simulink subsystem "Throttle_Map_2WD_NO_FILTER_NO_REGEN"  (R2023b)
settings: Solver=VariableStepAuto  StartTime=0.0  StopTime=10.0  RelTol=1e-3
undefined symbols (not defined in the file): tvs
settings Model: Creator=Inver  LastModifiedBy=Inver

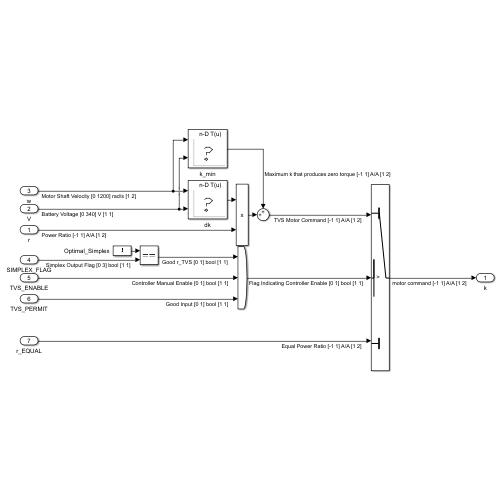
[thumbnail: Simulink's stored preview of the top-level diagram]
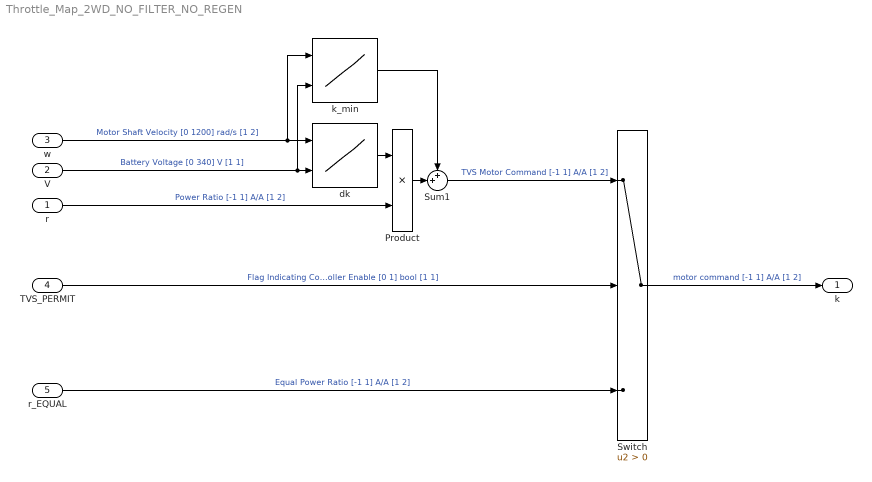
== system Throttle_Map_2WD_NO_FILTER_NO_REGEN ==
  r : Inport
  V : Inport  Port=2
  w : Inport  Port=3
  TVS_PERMIT : Inport  Port=4
  r_EQUAL : Inport  Port=5
  Product : Product
  Sum1 : Sum  Inputs=++|
  Switch : Switch  Criteria=u2 > Threshold  SaturateOnIntegerOverflow=off  InputSameDT=off
  dk : Lookup_n-D  LookupTableObject=''  BreakpointsForDimension1=tvs.motors.rpm_sweep_min  BreakpointsForDimension2=tvs.motors.voltage_sweep_min  BreakpointsForDimension1FirstPoint=10  BreakpointsForDimension2FirstPoint=10  BreakpointsForDimension1Spacing=12  BreakpointsForDimension2Spacing=12  IndexSearchMethod=Evenly spaced points  Table=tvs.motors.dk_grid  ExtrapMethod=Clip  DiagnosticForOutOfRangeInput=Error  InternalRulePriority=Speed  RndMeth=Simplest
      settings: InputPortMap=u0,u1
  k_min : Lookup_n-D  LookupTableObject=''  BreakpointsForDimension1=tvs.motors.rpm_sweep_min  BreakpointsForDimension2=tvs.motors.voltage_sweep_min  BreakpointsForDimension1FirstPoint=10  BreakpointsForDimension2FirstPoint=10  BreakpointsForDimension1Spacing=12  BreakpointsForDimension2Spacing=12  IndexSearchMethod=Evenly spaced points  Table=tvs.motors.k_grid_min  ExtrapMethod=Clip  DiagnosticForOutOfRangeInput=Error  InternalRulePriority=Speed  RndMeth=Simplest
      settings: InputPortMap=u0,u1
  k : Outport
  wires:
  w/1 -> dk/1, k_min/1  "Motor Shaft Velocity [0 1200] rad/s [1 2]"
  V/1 -> dk/2, k_min/2  "Battery Voltage [0 340] V [1 1]"
  r/1 -> Product/2  "Power Ratio [-1 1] A/A [1 2]"
  Sum1/1 -> Switch/1  "TVS Motor Command [-1 1] A/A [1 2]"
  k_min/1 -> Sum1/1
  dk/1 -> Product/1
  Product/1 -> Sum1/2
  Switch/1 -> k/1  "motor command [-1 1] A/A [1 2]"
  TVS_PERMIT/1 -> Switch/2  "Flag Indicating Controller Enable [0 1] bool [1 1]"
  r_EQUAL/1 -> Switch/3  "Equal Power Ratio [-1 1] A/A [1 2]"
